simulink model "Extended_Kalman"  (R2021a)
settings: Solver=VariableStepAuto  StartTime=0.0  StopTime=10.0  RelTol=1e-3
values from neighbouring files (symbols this model uses):
  g = 9.81    [Inverted_Pen.m]
  l = 2.5    [Inverted_Pen.m]
  m = 2    [Inverted_Pen.m]
  Q = 2e-4    (= 0.0002)    [Inverted_Pen.m]
  R = 2e-4    (= 0.0002)    [Inverted_Pen.m]
  Ts = 0.01    [Inverted_Pen.m]
libraries: simulink x2, sharedTrackingLibrary x1
settings Model: Creator=SOLONSO  LastModifiedBy=SOLONSO

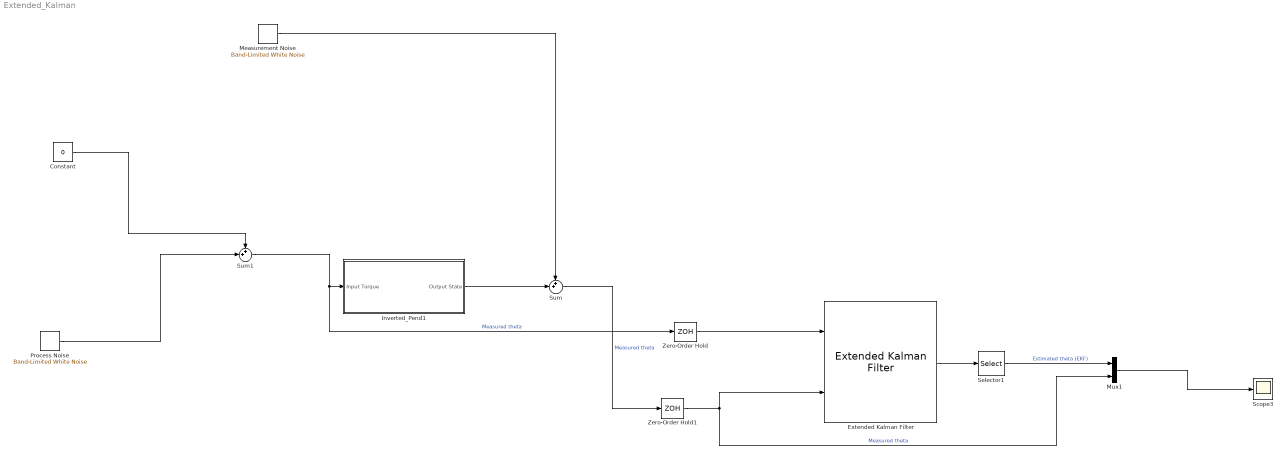
== system Extended_Kalman ==
  Constant : Constant  Value=0
  Extended Kalman Filter : sharedTrackingLibrary/Extended Kalman Filter  StateTransitionFcn=myStateTransitionFcn  HasStateTransitionJacobianFcn=off  HasAdditiveProcessNoise=Additive  ProcessNoise=diag([0 Q])  HasTimeVaryingProcessNoise=off  HasStateTransitionFcnExtraArgument=1  InitialState=x_0  InitialStateCovariance=1e-6  MeasurementFcn1=myMeasurementFcn  HasMeasurementJacobianFcn1=off  HasMeasurementEnablePort1=off  HasAdditiveMeasurementNoise1=Additive  MeasurementNoise1=R  HasTimeVaryingMeasurementNoise1=off  HasMeasurementFcnExtraArgument1=0  MeasurementFcn2=myMeasurementFcn  HasMeasurementJacobianFcn2=off  HasMeasurementEnablePort2=off  HasAdditiveMeasurementNoise2=Additive  MeasurementNoise2=1  HasTimeVaryingMeasurementNoise2=off  HasMeasurementFcnExtraArgument2=0  MeasurementFcn3=myMeasurementFcn  HasMeasurementJacobianFcn3=off  HasMeasurementEnablePort3=off  HasAdditiveMeasurementNoise3=Additive  MeasurementNoise3=1  HasTimeVaryingMeasurementNoise3=off  HasMeasurementFcnExtraArgument3=0  MeasurementFcn4=myMeasurementFcn  HasMeasurementJacobianFcn4=off  HasMeasurementEnablePort4=off  HasAdditiveMeasurementNoise4=Additive  MeasurementNoise4=1  HasTimeVaryingMeasurementNoise4=off  HasMeasurementFcnExtraArgument4=0  MeasurementFcn5=myMeasurementFcn  HasMeasurementJacobianFcn5=off  HasMeasurementEnablePort5=off  HasAdditiveMeasurementNoise5=Additive  MeasurementNoise5=1  HasTimeVaryingMeasurementNoise5=off  HasMeasurementFcnExtraArgument5=0  EnableMultirate=off  StateTransitionFcnSampleTime=1  MeasurementFcn1SampleTime=1  MeasurementFcn2SampleTime=1  MeasurementFcn3SampleTime=1  MeasurementFcn4SampleTime=1  MeasurementFcn5SampleTime=1  UseCurrentEstimator=on  OutputStateCovariance=off  DataType=double  SampleTime=Ts  NumberOfMeasurements=1
      settings: SourceProductBaseCode=CT,DR,TF,ID,LP,NV,AR,RO,RR,UV,VE
  Inverted_Pend1 : Subsystem
  Measurement Noise : simulink/Sources/Band-Limited White Noise  Cov=R*Ts  Ts=Ts  seed=[12347]
  Mux1 : Mux  Inputs=2
  Process Noise : simulink/Sources/Band-Limited White Noise  Cov=Q*Ts  Ts=Ts  seed=[23341]
  Scope3 : Scope
  Selector1 : Selector  InputPortWidth=2  IndexOptions=Index vector (dialog)  Indices=[1]  OutputSizes=1
  Sum : Sum  Inputs=++|
  Sum1 : Sum  Inputs=++|
  Zero-Order Hold : ZeroOrderHold  SampleTime=Ts
  Zero-Order Hold1 : ZeroOrderHold  SampleTime=Ts
  wires:
  Sum1/1 -> Zero-Order Hold/1, Inverted_Pend1/1(Input Torque)  "Measured theta"
  Mux1/1 -> Scope3/1
  Process Noise/1 -> Sum1/2
  Constant/1 -> Sum1/1
  Selector1/1 -> Mux1/1  "Estimated theta (EKF)"
  Extended Kalman Filter/1 -> Selector1/1
  Zero-Order Hold/1 -> Extended Kalman Filter/1
  Zero-Order Hold1/1 -> Mux1/2, Extended Kalman Filter/2  "Measured theta"
  Measurement Noise/1 -> Sum/1
  Sum/1 -> Zero-Order Hold1/1  "Measured theta"
  Inverted_Pend1/1(Output State) -> Sum/2

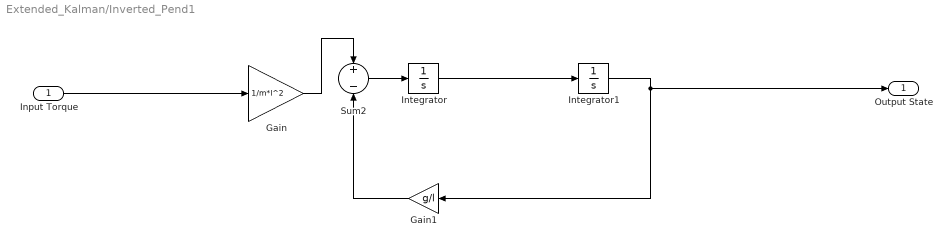
== system Extended_Kalman/Inverted_Pend1 ==
  Input Torque : Inport
  Gain : Gain  Gain=1/m*l^2
  Gain1 : Gain  Gain=g/l
  Integrator : Integrator
  Integrator1 : Integrator  InitialCondition=pi/18
  Sum2 : Sum  Inputs=+-
  Output State : Outport
  wires:
  Integrator1/1 -> Output State/1, Gain1/1
  Gain/1 -> Sum2/1
  Integrator/1 -> Integrator1/1
  Gain1/1 -> Sum2/2
  Sum2/1 -> Integrator/1
  Input Torque/1 -> Gain/1
